simulink model "untitled"  (R2023a)
settings: Solver=VariableStepAuto  StartTime=0.0  StopTime=10.0  RelTol=1e-3
values from neighbouring files (symbols this model uses):
  e = 0    [orb_elem.m]
  mi = (mi)    [orb_elem.m]
undefined symbols (not defined in the file or in its folder): Cd0, Cd1, drag, h0_ini, i0_ini, J2, J2_dist, l0, l1, m0, m1, man, ohm0_ini, omega_E, pcoRad, r0_dot_ini, r0_ini, Re, theta0_ini, x0_dot_ini, x0_ini, y0_dot_ini, y0_ini, z0_dot_ini, z0_ini
(part 2 of 2)

== matlab function untitled/ElemOrbLider ==
  data: mi input; ohm input; theta input; I input; x input; a1 output; y input; z input; x_dot input; y_dot input; z_dot input; e1 output; i1 output; Ohm1 output; omega1 output; f1 output; u1 output; L1 output; l1 output; omega_t1 output; lambda1 output; theta1 output; r0x_I output; r0y_I output; r0z_I output; r0_vec_I output; v0_vec_I output; r0_dotdot_vec input; a0_vec_I output; h0_vec_I output
function [a1,e1,i1,Ohm1,omega1,f1,u1,L1,l1,omega_t1,lambda1,theta1,r0x_I,r0y_I,r0z_I,r0_vec_I,v0_vec_I,a0_vec_I,h0_vec_I] = fcn(mi,ohm,theta,I,x,y,z,x_dot,y_dot,z_dot,r0_dotdot_vec)

[~,T_LVLH_In] = TransInerLVLH(ohm,theta,I);

r0_vec_I = T_LVLH_In*[x y z]';

r0x_I = r0_vec_I(1);
r0y_I = r0_vec_I(2);
r0z_I = r0_vec_I(3);

v0_vec_I = T_LVLH_In*[x_dot y_dot z_dot]';

a0_vec_I = T_LVLH_In*r0_dotdot_vec';

h0_vec_I = cross(r0_vec_I,v0_vec_I);

[a1,e1,i1,Ohm1,omega1,f1,u1,L1,l1,omega_t1,lambda1,theta1] = orb_elem(mi,r0_vec_I,v0_vec_I);

== matlab function untitled/ElemOrbLider1 ==
  data: mi input; ohm input; theta input; I input; x input; a0 output; y input; z input; x_dot input; y_dot input; z_dot input; e0 output; i0 output; Ohm0 output; omega0 output; f0 output; l0 output; omega_t0 output; lambda0 output; theta0 output; r0x_I output; r0y_I output; r0z_I output; r0_vec_I output; v0_vec_I output; h0_vec_I output; L0 output
function [a0,e0,i0,Ohm0,omega0,f0,l0,omega_t0,lambda0,theta0,r0x_I,r0y_I,r0z_I,r0_vec_I,v0_vec_I,h0_vec_I,L0] = fcn(mi,ohm,theta,I,x,y,z,x_dot,y_dot,z_dot)

[~,T_LVLH_In] = TransInerLVLH(ohm,theta,I);

r0_vec_I = T_LVLH_In*[x y z]';

r0x_I = r0_vec_I(1);
r0y_I = r0_vec_I(2);
r0z_I = r0_vec_I(3);

v0_vec_I = T_LVLH_In*[x_dot y_dot z_dot]';

h0_vec_I = cross(r0_vec_I,v0_vec_I);

[a0,e0,i0,Ohm0,omega0,f0,l0,omega_t0,lambda0,theta0,~,~] = orb_elem(mi,r0_vec_I,v0_vec_I);

%L0 = wrapTo2Pi(omega0 + Ohm0 + f0);
%L0 = wrapTo2Pi(omega0 + Ohm0);
L0 = wrapTo2Pi(Ohm0);
